simulink library "gaussianProcess_ul"  (R2018b)
settings: Solver=VariableStepAuto  StartTime=0.0  StopTime=10.0  RelTol=1e-3
settings Model: Creator=asiddiq2  LastModifiedBy=asiddiq2

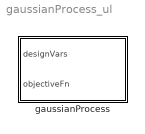
== system gaussianProcess_ul ==
  gaussianProcess : Subsystem  mask{dt=1}
      mask prompts: dt "Sampling time interval"

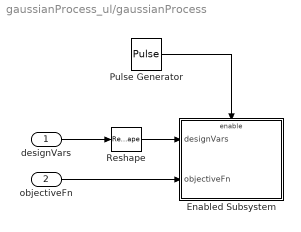
== system gaussianProcess_ul/gaussianProcess ==
  designVars : Inport
  objectiveFn : Inport  Port=2
  Enabled Subsystem : Subsystem  TreatAsAtomicUnit=on
  Pulse Generator : DiscretePulseGenerator  PulseType=Time based  Period=dt  PulseWidth=5
  Reshape : Reshape  OutputDimensionality=Column vector (2-D)
  wires:
  designVars/1 -> Reshape/1
  objectiveFn/1 -> Enabled Subsystem/2(objectiveFn)
  Pulse Generator/1 -> Enabled Subsystem/Enable
  Reshape/1 -> Enabled Subsystem/1(designVars)

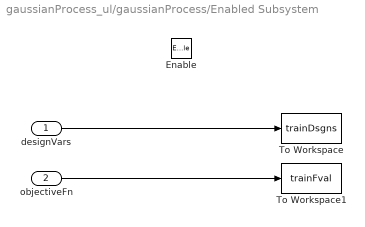
== system gaussianProcess_ul/gaussianProcess/Enabled Subsystem ==
  designVars : Inport
  objectiveFn : Inport  Port=2
  Enable : EnablePort
  To Workspace : ToWorkspace  VariableName=trainDsgns  SaveFormat=Timeseries  SampleTime=-1
  To Workspace1 : ToWorkspace  VariableName=trainFval  SaveFormat=Timeseries  SampleTime=-1
  wires:
  objectiveFn/1 -> To Workspace1/1
  designVars/1 -> To Workspace/1
